simulink model "halfadderdesign"  (R2014a)
settings: Solver=ode45  StartTime=0.0  StopTime=10.0  RelTol=1e-3
settings Model: Creator=Andrew  LastModifiedBy=Andrew

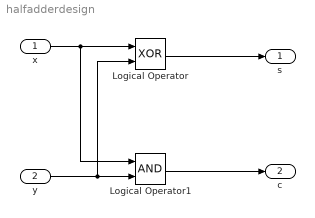
== system halfadderdesign ==
  x : Inport
  y : Inport  Port=2
  Logical Operator : Logic  Operator=XOR  AllPortsSameDT=off  OutDataTypeStr=boolean
  Logical Operator1 : Logic  AllPortsSameDT=off  OutDataTypeStr=boolean
  s : Outport
  c : Outport  Port=2
  wires:
  x/1 -> Logical Operator1/1, Logical Operator/1
  y/1 -> Logical Operator/2, Logical Operator1/2
  Logical Operator/1 -> s/1
  Logical Operator1/1 -> c/1
